simulink model "lab3_open_loop"  (R2023a)
settings: Solver=VariableStepAuto  StartTime=0.0  StopTime=8  RelTol=1e-3
values from neighbouring files (symbols this model uses):
  anum = 0.3    [lab3.m]
  den = [1 0 w0^2]    [lab3.m]
  denD = cell2mat(denD)    [lab3.m]
  num = G*w0^2    (= 4)    [lab3.m]
  numD = cell2mat(numD)    [lab3.m]
settings Model: Creator=dgkegkas2023  LastModifiedBy=dgkegkas2023

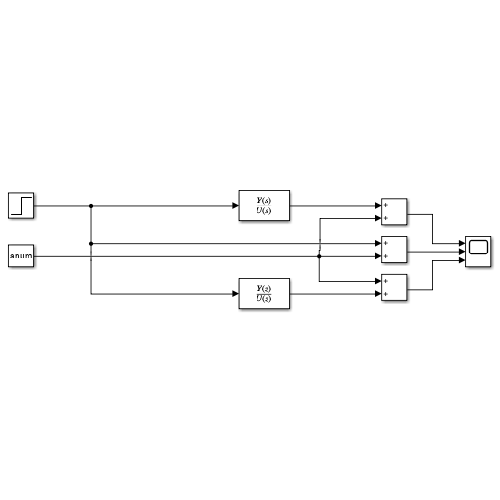
[thumbnail: Simulink's stored preview of the top-level diagram]
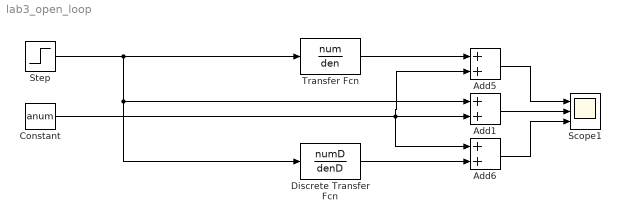
== system lab3_open_loop ==
  Add1 : Sum
  Add5 : Sum
  Add6 : Sum
  Constant : Constant  Value=anum
  Discrete Transfer Fcn : DiscreteTransferFcn  Numerator=numD  Denominator=denD
  Scope1 : Scope  NumInputPorts=3
  Step : Step  After=0.05  SampleTime=0.1
  Transfer Fcn : TransferFcn  Numerator=num  Denominator=den
  wires:
  Step/1 -> Add1/1, Discrete Transfer Fcn/1, Transfer Fcn/1
  Constant/1 -> Add6/1, Add5/2, Add1/2
  Discrete Transfer Fcn/1 -> Add6/2
  Add5/1 -> Scope1/1
  Add6/1 -> Scope1/3
  Transfer Fcn/1 -> Add5/1
  Add1/1 -> Scope1/2
